simulink model "test_NetworkInterface_TCP_InputOutput"  (R2016b)
settings: Solver=FixedStepDiscrete  StartTime=0.0  StopTime=inf  FixedStep=0.05  RelTol=1e-3
libraries: LIB_NetwokInterface x1
settings Model: SimulationMode=external  ExtModeTrigDuration=10000  Creator=constantin  LastModifiedBy=valtin
settings DataIOCC: LimitDataPoints=on  SaveFormat=Array
settings OptimizationCC: ExpressionDepthLimit=2147483647  LifeSpan=1
settings DebuggingCC: UnderspecifiedInitializationDetection=Classic  MergeDetectMultiDrivingBlocksExec=none  SolverPrmCheckMsg=warning  StateNameClashWarn=warning  SFUnexpectedBacktrackingDiag=warning  SFNoUnconditionalDefaultTransitionDiag=warning  SFExecutionAtInitializationDiag=none
settings HardwareCC: ProdBitPerPointer=32  ProdBitPerSizeT=32  ProdBitPerPtrDiffT=32  ProdLargestAtomicFloat=None  ProdIntDivRoundTo=Undefined  ProdEndianess=Unspecified  ProdWordSize=32  ProdHWDeviceType=32-bit Generic
settings ModelReferenceCC: PropagateSignalLabelsOutOfModel=off
settings SFSimCC: SimParseCustomCode=off
settings RTWCC: SystemTargetFile=ert_linux.tlc  MakeCommand=make_rtw OPTS=-DWITH_HW OPTIMIZATION_FLAGS=-O3  TemplateMakefile=ert_linux.tmf  Description=Linux Embedded Coder  TargetLang=C++
settings CodeAppCC: IgnoreCustomStorageClasses=off  CustomSymbolStrType=$N$R$M  InternalIdentifier=Classic
settings STFCustomTargetCC: ModelReferenceCompliant=off  GeneratePreprocessorConditionals=Disable all  CombineOutputUpdateFcns=on  ERTCustomFileBanners=on  SupportComplex=off  RemoveResetFunc=on  SupportVariableSizeSignals=on  MATLABClassNameForMDSCustomization=Simulink.SoftwareTarget.ERTCustomization  GRTInterface=off  SystemTargetFile=ert_linux.tlc
settings ERTTargetCC: ModelReferenceCompliant=off  ParMdlRefBuildCompliant=off  CompOptLevelCompliant=off  ConcurrentExecutionCompliant=off  GeneratePreprocessorConditionals=Disable all  ERTFirstTimeCompliant=off  SupportComplex=off  SupportContinuousTime=on  SupportNonInlinedSFcns=on  SupportVariableSizeSignals=on  ModelStepFunctionPrototypeControlCompliant=off  CPPClassGenCompliant=off  UseToolchainInfoCompliant=off  ExtMode=on  MultiInstanceErrorCode=None  ERTCustomFileTemplate=ert_linux_file_process.tlc  ConvertIfToSwitch=off  SuppressUnreachableDefaultCases=off
settings ConfigComp: CovMetricSettings=dw  CovHtmlReporting=on  CovSaveCumulativeToWorkspaceVar=on  CovSaveSingleToWorkspaceVar=on  CovExternalEMLEnable=off  CovSFcnEnable=off
settings ConfigurationSet: Description=SimMechanics 2G

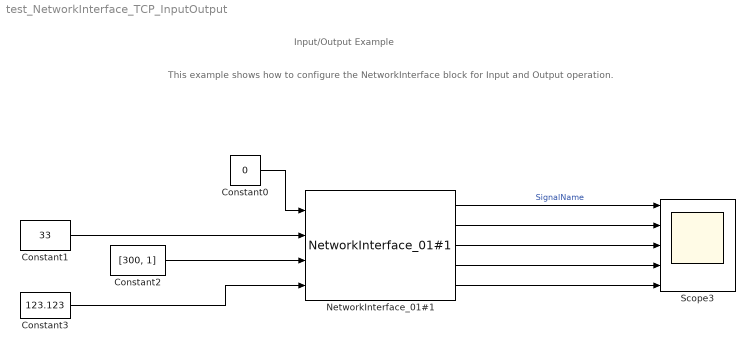
== system test_NetworkInterface_TCP_InputOutput ==
  note: This example shows how to configure the NetworkInterface block for Input and Output operation.
  note: Input/Output Example
  Constant0 : Constant  Value=0  OutDataTypeStr=double  SampleTime=-1
  Constant1 : Constant  Value=33  OutDataTypeStr=double  SampleTime=-1
  Constant2 : Constant  Value=[300, 1]  OutDataTypeStr=double  SampleTime=-1
  Constant3 : Constant  Value=123.123  OutDataTypeStr=double  SampleTime=-1
  NetworkInterface_01#1 : LIB_NetwokInterface/NetworkInterface_01#1  inputs=[1,2,1]  outputs=[1,2,2,1]  initialOutputValues=1  SampleTime=-1  useUDP=off  startConnection=on  localPort=20000  remoteIP='127.0.0.1'  remotePort=20001
  Scope3 : Scope  NumInputPorts=5
  wires:
  NetworkInterface_01#1/1 -> Scope3/1  "SignalName"
  NetworkInterface_01#1/2 -> Scope3/2
  Constant1/1 -> NetworkInterface_01#1/2
  Constant2/1 -> NetworkInterface_01#1/3
  Constant3/1 -> NetworkInterface_01#1/4
  Constant0/1 -> NetworkInterface_01#1/1
  NetworkInterface_01#1/3 -> Scope3/3
  NetworkInterface_01#1/4 -> Scope3/4
  NetworkInterface_01#1/5 -> Scope3/5
